simulink model "if_else_testing"  (R2023b)
settings: Solver=VariableStepAuto  StartTime=0.0  StopTime=0.1  RelTol=1e-3
settings Model: Creator=alfre  LastModifiedBy=alfre

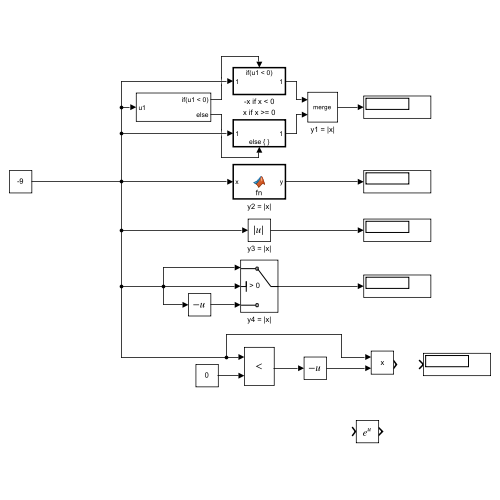
[thumbnail: Simulink's stored preview of the top-level diagram]
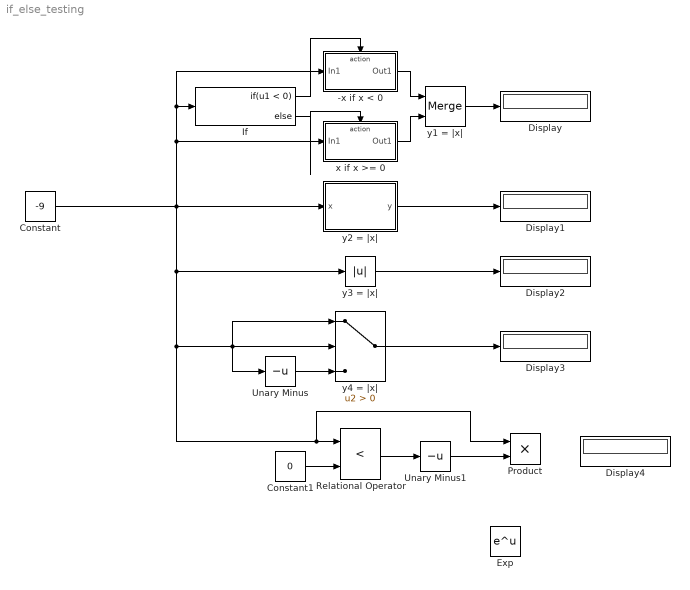
== system if_else_testing ==
  -x if x < 0 : Subsystem  TreatAsAtomicUnit=on
  Constant : Constant  Value=-9
  Constant1 : Constant  Value=0
  Display{,1..4} (5 alike) : Display
  Exp : Math
  If : If  IfExpression=u1 < 0
  Product : Product
  Relational Operator : RelationalOperator  Operator=<  OutDataTypeStr=boolean  RndMeth=Simplest  InputSameDT=off
  Unary Minus : UnaryMinus
  Unary Minus1 : UnaryMinus
  x if x >= 0 : Subsystem  TreatAsAtomicUnit=on
  y1 = |x| : Merge
  y2 = |x| : MATLAB Function  TreatAsAtomicUnit=on
  y3 = |x| : Abs  SaturateOnIntegerOverflow=off
  y4 = |x| : Switch  Criteria=u2 > Threshold  SaturateOnIntegerOverflow=off  InputSameDT=off
  wires:
  Constant/1 -> Product/1, Relational Operator/1, Unary Minus/1, y4 = |x|/1, y4 = |x|/2, y3 = |x|/1, y2 = |x|/1(x), If/1, -x if x < 0/1(In1), x if x >= 0/1(In1)
  If/1 -> -x if x < 0/Action
  If/2 -> x if x >= 0/Action
  -x if x < 0/1(Out1) -> y1 = |x|/1
  x if x >= 0/1(Out1) -> y1 = |x|/2
  y1 = |x|/1 -> Display/1
  y2 = |x|/1(y) -> Display1/1
  y3 = |x|/1 -> Display2/1
  y4 = |x|/1 -> Display3/1
  Unary Minus/1 -> y4 = |x|/3
  Constant1/1 -> Relational Operator/2
  Relational Operator/1 -> Unary Minus1/1
  Unary Minus1/1 -> Product/2

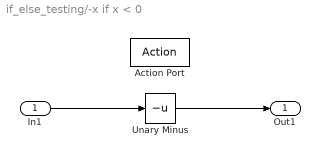
== system if_else_testing/-x if x < 0 ==
  In1 : Inport
  Action Port : ActionPort  ActionPortLabel=if(u1 < 0)
  Unary Minus : UnaryMinus
  Out1 : Outport
  wires:
  In1/1 -> Unary Minus/1
  Unary Minus/1 -> Out1/1

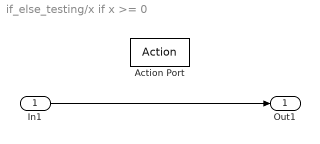
== system if_else_testing/x if x >= 0 ==
  In1 : Inport
  Action Port : ActionPort  ActionPortLabel=else
  Out1 : Outport
  wires:
  In1/1 -> Out1/1

== matlab function if_else_testing/y2 = |x| ==
  data: x input; y output
function y = fn(x)
y = x * (-1)^(x < 0);
% Other options:
% -------------------
% if x < 0, y = -x;
% else,     y = x;
% end
% -------------------
% if x < 0
%     y = -x;
% else
%     y = x;
% end
% -------------------
